simulink model "IRGLMHybridController"  (R2022b)
settings: Solver=FixedStepAuto  StartTime=0.0  StopTime=1E6  FixedStep=1/2000  RelTol=1e-3
undefined symbols (not defined in the file): Pull, up
libraries: cstblocks x7, speedgoatlib_IO183 x5, slrealtimeutilitieslib x2, slrealtimeiplib x2, dspstat3 x1
settings Model: Creator=MOSA  LastModifiedBy=MOSA
settings SolverCC: ConcurrentTasks=on  PositivePriorityOrder=on
settings OptimizationCC: BlockReduction=off  OptimizeBlockIOStorage=off
settings DebuggingCC: TasksWithSamePriorityMsg=none
settings HardwareCC: ProdBitPerLong=64  ProdLongLongMode=on  ProdHWDeviceType=Intel->x86-64 (Linux 64)
settings RTWCC: Description=Simulink Real-Time  SystemTargetFile=slrealtime.tlc  TemplateMakefile=slrealtime_default_tmf  Toolchain=Simulink Real-Time Toolchain  BuildConfiguration=Faster Runs  CodeExecutionProfiling=on  TargetLang=C++

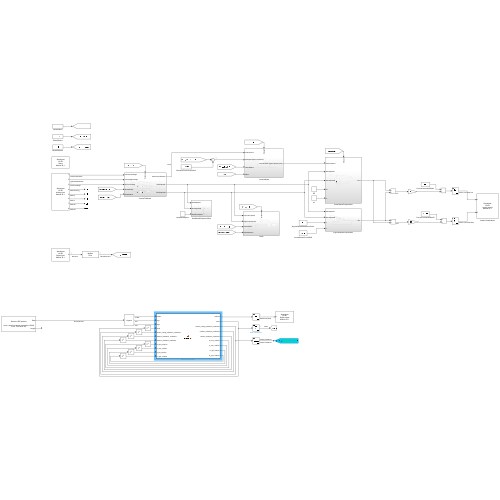
[thumbnail: Simulink's stored preview of the top-level diagram]
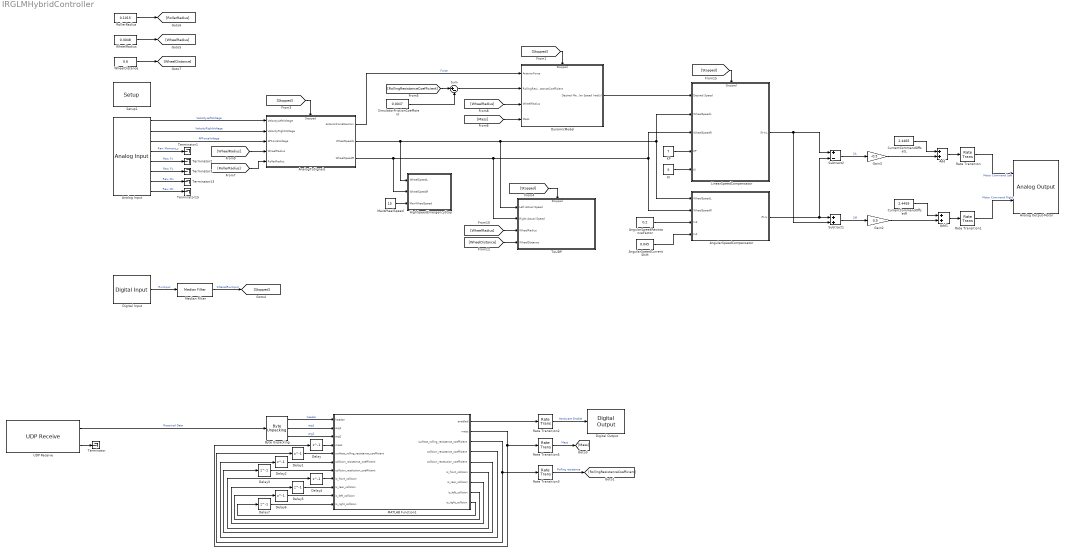
== system IRGLMHybridController ==
  Add : Sum
  Add1 : Sum
  Analog Input : speedgoatlib_IO183/Analog Input  Priority=0  parModuleId=1  parSampTime=1/2000  parPciSlot=-1  parAdChannelLow=1  parAdChannelHigh=8
      settings: SourceProductName=Simulink Real-Time: Speedgoat I/O Blockset
  Analog Output-Motor : speedgoatlib_IO183/Analog Output  parModuleId=1  parSampTime=-1  parDaSimult=on  parPciSlot=-1  parDaChannels=[1 2]  parDaInit=[0 0 0 0]  parDaReset=[1 1 1 1]
      settings: SourceProductName=Simulink Real-Time: Speedgoat I/O Blockset
  AnalogToSignals : Subsystem
      settings: PortSchema="{\"entries\":[{\"content\":{\"sides\":[{\"content\":{\"connectorIds\":[\"In1\",\"In2\",\"In3\",\"In4\",\"In5\"]},\"type\":\"ConnectorPlacement.EquallySpacedRectSide\",\"uuid\":\"33d34f65-8288-4f26-a259-c6a495dc8706\"},{\"content\":{\"connectorIds\":[\"Out1\",\"Out2\",\"Out3\"],\"side\":\"RIGHT\"},\"type\":\"ConnectorPlacement.EquallySpacedRectSide\",\"uuid\":\"464c1a73-e25a-412b-b070-c0497a01c93b\"},{\"content\":{\"connectorIds\":[\"In6\"],\"side\":\"TOP\"},\"type\":\"ConnectorPlacement.EquallySpacedRectSide\",\"uuid\":\"eb57de37-2540-4fa6-8c21-04ed7dfe5e59\"}]},\"type\":\"ConnectorPlacement.EquallySpacedConnector\",\"uuid\":\"7b998d75-753a-4c6e-bb60-3204e0b4afb9\"}],\"packageUris\":[\"http://schema.mathworks.com/mf0/Connector/R2020b\"],\"version\":\"1.0\"}"
  AngularSpeedCompensator : Subsystem
  AngularSpeedCurrentShift : Constant  Value=0.045
  AngularSpeedResistanceFactor : Constant  Value=0.2
  Byte Unpacking : slrealtimeutilitieslib/Byte Unpacking  MaskUnpackedDataTypes={['uint32'],['double'],['double']}  MaskUnpackedDataSizes={[1] [1] [1]}  MaskAlignment=4
  CurrentCommandOffsetL : Constant  Value=2.4465
  CurrentCommandOffsetR : Constant  Value=2.4459
  Delay{,1..7} (8 alike) : Delay  DelayLength=1  InitialCondition=0
  Digital Input : speedgoatlib_IO183/Digital Input  parModuleId=1  parSampTime=1/2000  parPciSlot=-1  parDiChannels=2
      settings: SourceProductName=Simulink Real-Time: Speedgoat I/O Blockset
  Digital Output : speedgoatlib_IO183/Digital Output  parModuleId=1  parSampTime=-1  parPciSlot=-1  parDoChannels=1  parDoInit=0  parDoReset=1
      settings: SourceProductName=Simulink Real-Time: Speedgoat I/O Blockset
  DynamicModel : Subsystem
      settings: PortSchema="{\"entries\":[{\"content\":{\"sides\":[{\"content\":{\"connectorIds\":[\"In1\",\"In2\",\"In3\",\"In4\"]},\"type\":\"ConnectorPlacement.EquallySpacedRectSide\",\"uuid\":\"698b5f1b-e41d-47ec-8a78-8e111d48540c\"},{\"content\":{\"connectorIds\":[\"Out1\"],\"side\":\"RIGHT\"},\"type\":\"ConnectorPlacement.EquallySpacedRectSide\",\"uuid\":\"a52a2d34-ec8e-4f9e-8684-ea9d86dd283b\"},{\"content\":{\"connectorIds\":[\"In5\"],\"side\":\"TOP\"},\"type\":\"ConnectorPlacement.EquallySpacedRectSide\",\"uuid\":\"faf14a61-efdc-45c6-85a8-2f82d0ccb291\"}]},\"type\":\"ConnectorPlacement.EquallySpacedConnector\",\"uuid\":\"7a7495df-049f-4dbe-8bcc-a94b4d420872\"}],\"packageUris\":[\"http://schema.mathworks.com/mf0/Connector/R2020b\"],\"version\":\"1.0\"}"
  Gain2 : Gain  Gain=0.5
  Gain3 : Gain  Gain=-0.5
  HighSpeedEmergencyStop : Subsystem
  KI : Constant  Value=5
  KP : Constant  Value=7
  LinearSpeedCompensator : Subsystem
      settings: PortSchema="{\"entries\":[{\"content\":{\"sides\":[{\"content\":{\"connectorIds\":[\"In1\",\"In2\",\"In3\",\"In4\",\"In5\"]},\"type\":\"ConnectorPlacement.EquallySpacedRectSide\",\"uuid\":\"9b7edc03-5e72-48f4-bed7-21920e73c297\"},{\"content\":{\"connectorIds\":[\"Out1\"],\"side\":\"RIGHT\"},\"type\":\"ConnectorPlacement.EquallySpacedRectSide\",\"uuid\":\"1856f1b7-fc85-471c-9138-bfce3ff137ef\"},{\"content\":{\"connectorIds\":[\"In6\"],\"side\":\"TOP\"},\"type\":\"ConnectorPlacement.EquallySpacedRectSide\",\"uuid\":\"701dcd4a-e839-44a9-b16d-b7c230713f8d\"}]},\"type\":\"ConnectorPlacement.EquallySpacedConnector\",\"uuid\":\"564dc47d-1095-4697-b7b0-537dc9d65b40\"}],\"packageUris\":[\"http://schema.mathworks.com/mf0/Connector/R2020b\"],\"version\":\"1.0\"}"
  MATLAB Function1 : MATLAB Function  TreatAsAtomicUnit=on
  MaxWheelSpeed : Constant  Value=15
  Median Filter : dspstat3/Median Filter  WindowLength=5  SimulateUsing=Interpreted execution
      settings: LibrarySourceBlock=|
      | dspfdesign/Median
      | Filter
  Rate Transition : RateTransition
  Rate Transition1 : RateTransition
  Rate Transition2 : RateTransition  OutPortSampleTime=1/2000
  Rate Transition3 : RateTransition  OutPortSampleTime=1/2000
  Rate Transition5 : RateTransition  OutPortSampleTime=1/2000
  RollerRadius : Constant  Value=0.1015
  Setup1 : speedgoatlib_IO183/Setup  parModuleId=1  parPciSlot=-1  parDaSimult=on  parAdCoupling=Single Ended  parAdRange=+-10V  parAdChannelLow=1  parAdChannelHigh=8  parDaChannels=[1:2]  parDaRange=0..5V  parDaInit=[0]  parDaReset=[1]  parDoChannels=[1]  parDoInit=[0]  parDoReset=[1]  parDiChannels=[2]  parIOPullReferenceFront=Pull-up (3.3V)  parIOPullReferenceRear=Pull-up (3.3V)
      settings: SourceProductName=Simulink Real-Time: Speedgoat I/O Blockset
  SimulatorFrictionCoefficient : Constant  Value=0.0047
  Subtract1 : Sum
  Subtract2 : Sum  Inputs=+-
  Sum : Sum  Inputs=|+-
  Terminator{,1..3,13,15} (6 alike) : Terminator
  ToUDP : Subsystem
      settings: PortSchema="{\"entries\":[{\"content\":{\"sides\":[{\"content\":{\"connectorIds\":[\"In1\",\"In2\",\"In3\",\"In4\"]},\"type\":\"ConnectorPlacement.EquallySpacedRectSide\",\"uuid\":\"20cbcfc2-0ca7-4a2f-a613-0278f24034ac\"},{\"content\":{\"connectorIds\":[],\"side\":\"RIGHT\"},\"type\":\"ConnectorPlacement.EquallySpacedRectSide\",\"uuid\":\"dd88a308-46d9-424c-b176-6f22faf13019\"},{\"content\":{\"connectorIds\":[\"In5\"],\"side\":\"TOP\"},\"type\":\"ConnectorPlacement.EquallySpacedRectSide\",\"uuid\":\"69795427-50da-496d-bb46-4af6bccb20c3\"},{\"content\":{\"connectorIds\":[],\"side\":\"BOTTOM\"},\"type\":\"ConnectorPlacement.EquallySpacedRectSide\",\"uuid\":\"b34d6e53-d8ac-4a7b-a484-2036578c791d\"}]},\"type\":\"ConnectorPlacement.EquallySpacedConnector\",\"uuid\":\"611fc7d8-fafd-42e7-a535-d43e2501456a\"}],\"packageUris\":[\"http://schema.mathworks.com/mf0/Connector/R2020b\"],\"version\":\"1.0\"}"
  UDP Receive : slrealtimeiplib/UDP Receive  useHostTargetConn=on  ipAddress=192.168.0.200  localPort=25000  rcvWidth=20  rcvFmAny=off  fmAddress=192.168.0.159  sampleTime=1/200  enableMessage=off  maxPackets=1
  WheelDistance : Constant  Value=0.6
  WheelRadius : Constant  Value=0.3048
  wires:
  KI/1 -> LinearSpeedCompensator/5(KI)
  [Stopped] -> ToUDP/5(Stopped)
  [RollingResistanceCoefficient] -> Sum/1
  Subtract1/1 -> Gain2/1  "2iR"
  Sum/1 -> DynamicModel/2(RollingResistanceCoefficient)
  Gain3/1 -> Add/2
  Gain2/1 -> Add1/2
  Analog Input/5 -> Terminator2/1  "Raw Fx"
  Rate Transition1/1 -> Analog Output-Motor/2  "Motor Command Right"
  DynamicModel/1(Desired Mean Angular Speed (rad/s)) -> LinearSpeedCompensator/1(Desired Speed)
  KP/1 -> LinearSpeedCompensator/4(KP)
  [Stopped] -> LinearSpeedCompensator/6(Stopped)
  LinearSpeedCompensator/1(iR+iL) -> Subtract2/1, Subtract1/2
  UDP Receive/1 -> Byte Unpacking/1  "Received Data"
  Rate Transition2/1 -> Digital Output/1  "Hardware Enable"
  Digital Input/1 -> Median Filter/1  "RunInput"
  SimulatorFrictionCoefficient/1 -> Sum/2
  Analog Input/4 -> Terminator1/1  "Raw Moment_y"
  Median Filter/1 -> [Stopped]  "FilteredRunInput"
  Analog Input/7 -> Terminator13/1  "Raw Mx"
  Analog Input/6 -> Terminator3/1  "Raw Fy"
  Analog Input/8 -> Terminator15/1  "Raw Mz"
  UDP Receive/2 -> Terminator/1
  AnalogToSignals/1(AnteriorForceNewton) -> DynamicModel/1("AnteriorForce ")  "Force"
  Rate Transition/1 -> Analog Output-Motor/1  "Motor Command Left"
  Subtract2/1 -> Gain3/1  "2iL"
  Add/1 -> Rate Transition/1
  CurrentCommandOffsetR/1 -> Add1/1
  Rate Transition5/1 -> [Mass]  "Mass"
  Rate Transition3/1 -> [RollingResistanceCoefficient]  "Rolling resistance"
  CurrentCommandOffsetL/1 -> Add/1
  Add1/1 -> Rate Transition1/1
  [Mass] -> DynamicModel/4(Mass)
  WheelRadius/1 -> [WheelRadius]
  [WheelDistance] -> ToUDP/4(WheelDistance)
  RollerRadius/1 -> [RollerRadius]
  [WheelRadius] -> DynamicModel/3(WheelRadius)
  [WheelRadius] -> ToUDP/3(WheelRadius)
  WheelDistance/1 -> [WheelDistance]
  AnalogToSignals/2(WheelSpeedL) -> HighSpeedEmergencyStop/1(WheelSpeedL), AngularSpeedCompensator/1(WheelSpeedL), LinearSpeedCompensator/2(WheelSpeedL), ToUDP/1(Left Actual Speed)
  AnalogToSignals/3(WheelSpeedR) -> HighSpeedEmergencyStop/2(WheelSpeedR), LinearSpeedCompensator/3(WheelSpeedR), AngularSpeedCompensator/2(WheelSpeedR), ToUDP/2(Right Actual Speed)
  Analog Input/1 -> AnalogToSignals/1(VelocityLeftVoltage)  "VelocityLeftVoltage"
  Analog Input/2 -> AnalogToSignals/2(VelocityRightVoltage)  "VelocityRightVoltage"
  Analog Input/3 -> AnalogToSignals/3(APForceVoltage)  "APForceVoltage"
  [WheelRadius] -> AnalogToSignals/4(WheelRadius)
  [RollerRadius] -> AnalogToSignals/5(RollerRadius)
  [Stopped] -> AnalogToSignals/6(Stopped)
  [Stopped] -> DynamicModel/5(Stopped)
  MaxWheelSpeed/1 -> HighSpeedEmergencyStop/3(MaxWheelSpeed)
  AngularSpeedCompensator/1(iR-iL) -> Subtract1/1, Subtract2/2
  AngularSpeedResistanceFactor/1 -> AngularSpeedCompensator/3(In3)
  AngularSpeedCurrentShift/1 -> AngularSpeedCompensator/4(In4)
  Byte Unpacking/1 -> MATLAB Function1/1(header)  "header"
  Byte Unpacking/2 -> MATLAB Function1/2(arg1)  "arg1"
  Byte Unpacking/3 -> MATLAB Function1/3(arg2)  "arg2"
  MATLAB Function1/1(enabled) -> Rate Transition2/1
  MATLAB Function1/9(is_right_collision) -> Delay7/1
  MATLAB Function1/8(is_left_collision) -> Delay6/1
  MATLAB Function1/7(is_rear_collision) -> Delay5/1
  MATLAB Function1/6(is_front_collision) -> Delay4/1
  MATLAB Function1/5(collision_restitution_coefficient) -> Delay3/1
  MATLAB Function1/4(collision_resistance_coefficient) -> Delay2/1
  MATLAB Function1/3(surface_rolling_resistance_coefficient) -> Rate Transition3/1, Delay1/1
  MATLAB Function1/2(mass) -> Rate Transition5/1, Delay/1
  Delay/1 -> MATLAB Function1/4("mass ")
  Delay1/1 -> MATLAB Function1/5("surface_rolling_resistance_coefficient ")
  Delay2/1 -> MATLAB Function1/6("collision_resistance_coefficient ")
  Delay3/1 -> MATLAB Function1/7("collision_restitution_coefficient ")
  Delay4/1 -> MATLAB Function1/8("is_front_collision ")
  Delay5/1 -> MATLAB Function1/9("is_rear_collision ")
  Delay6/1 -> MATLAB Function1/10("is_left_collision ")
  Delay7/1 -> MATLAB Function1/11("is_right_collision ")

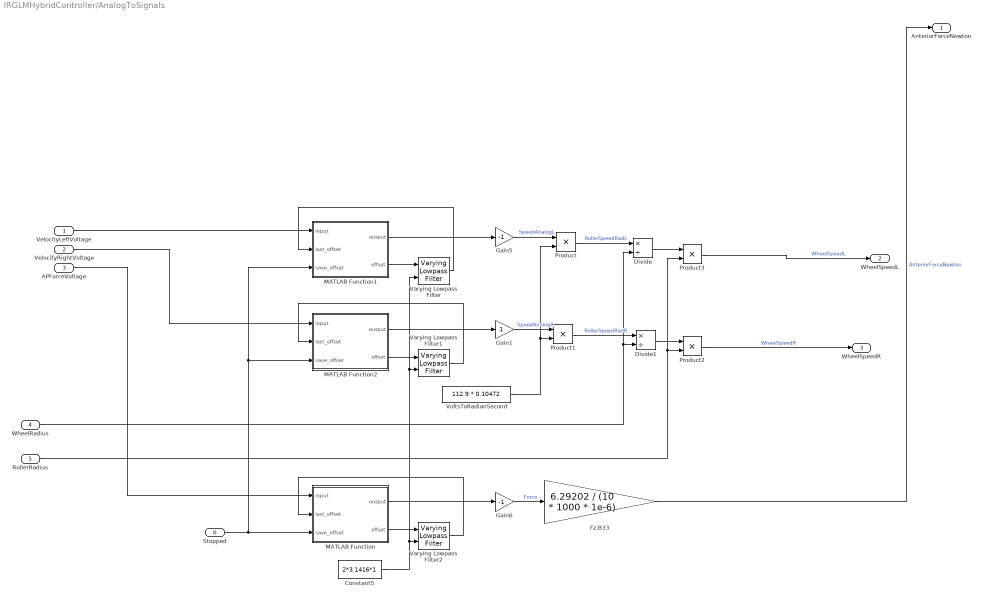
== system IRGLMHybridController/AnalogToSignals ==
  VelocityLeftVoltage : Inport
  VelocityRightVoltage : Inport  Port=2
  APForceVoltage : Inport  Port=3
  WheelRadius : Inport  Port=4
  RollerRadius : Inport  Port=5
  Stopped : Inport  Port=6
  Constant5 : Constant  Value=2*3.1416*1
  Divide : Product  Inputs=*/
  Divide1 : Product  Inputs=*/
  Fz.B33 : Gain  Gain="6.29202 / (10 * 1000  * 1e-6)"
  Gain1 : Gain
  Gain5 : Gain  Gain=-1
  Gain6 : Gain  Gain=-1
  MATLAB Function : MATLAB Function  TreatAsAtomicUnit=on
  MATLAB Function1 : MATLAB Function  TreatAsAtomicUnit=on
  MATLAB Function2 : MATLAB Function  TreatAsAtomicUnit=on
  Product{,1..3} (4 alike) : Product
  Varying Lowpass Filter : cstblocks/Linear Parameter Varying/Varying Lowpass Filter  N=1
  Varying Lowpass Filter1 : cstblocks/Linear Parameter Varying/Varying Lowpass Filter  N=1
  Varying Lowpass Filter2 : cstblocks/Linear Parameter Varying/Varying Lowpass Filter  N=1
  VoltsToRadianSecond : Constant  Value=112.9 * 0.10472
  AnteriorForceNewton : Outport
  WheelSpeedL : Outport  Port=2
  WheelSpeedR : Outport  Port=3
  wires:
  VelocityLeftVoltage/1 -> MATLAB Function1/1(input)
  Stopped/1 -> MATLAB Function1/3(save_offset), MATLAB Function2/3(save_offset), MATLAB Function/3(save_offset)
  WheelRadius/1 -> Divide/2, Divide1/2
  Gain5/1 -> Product/1  "SpeedAnalogL"
  Product2/1 -> WheelSpeedR/1  "WheelSpeedR"
  MATLAB Function1/2(offset) -> Varying Lowpass Filter/1
  Constant5/1 -> Varying Lowpass Filter/2, Varying Lowpass Filter1/2, Varying Lowpass Filter2/2
  Varying Lowpass Filter1/1 -> MATLAB Function2/2(last_offset)
  Product3/1 -> WheelSpeedL/1  "WheelSpeedL"
  Varying Lowpass Filter/1 -> MATLAB Function1/2(last_offset)
  RollerRadius/1 -> Product3/2, Product2/2
  VoltsToRadianSecond/1 -> Product/2, Product1/2
  MATLAB Function1/1(output) -> Gain5/1
  MATLAB Function2/1(output) -> Gain1/1
  Product1/1 -> Divide1/1  "RollerSpeedRadR"
  Gain1/1 -> Product1/1  "SpeedAnalogR"
  Product/1 -> Divide/1  "RollerSpeedRadL"
  MATLAB Function2/2(offset) -> Varying Lowpass Filter1/1
  MATLAB Function/1(output) -> Gain6/1
  Gain6/1 -> Fz.B33/1  "Force"
  MATLAB Function/2(offset) -> Varying Lowpass Filter2/1
  Divide1/1 -> Product2/1
  Fz.B33/1 -> AnteriorForceNewton/1  "AnteriorForceNewton"
  Divide/1 -> Product3/1
  APForceVoltage/1 -> MATLAB Function/1(input)
  Varying Lowpass Filter2/1 -> MATLAB Function/2(last_offset)
  VelocityRightVoltage/1 -> MATLAB Function2/1(input)

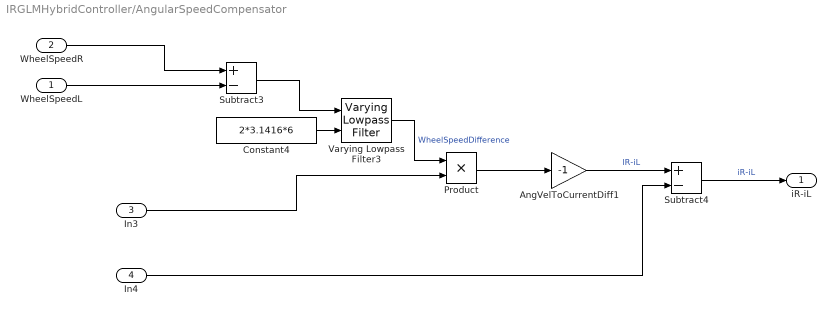
== system IRGLMHybridController/AngularSpeedCompensator ==
  WheelSpeedL : Inport
  WheelSpeedR : Inport  Port=2
  In3 : Inport  Port=3
  In4 : Inport  Port=4
  AngVelToCurrentDiff1 : Gain  Gain=-1
  Constant4 : Constant  Value=2*3.1416*6
  Product : Product
  Subtract3 : Sum  Inputs=+-
  Subtract4 : Sum  Inputs=+-
  Varying Lowpass Filter3 : cstblocks/Linear Parameter Varying/Varying Lowpass Filter  N=2
  iR-iL : Outport
  wires:
  Varying Lowpass Filter3/1 -> Product/1  "WheelSpeedDifference"
  Subtract3/1 -> Varying Lowpass Filter3/1
  AngVelToCurrentDiff1/1 -> Subtract4/1  "lR-iL"
  In3/1 -> Product/2
  Constant4/1 -> Varying Lowpass Filter3/2
  Product/1 -> AngVelToCurrentDiff1/1
  WheelSpeedL/1 -> Subtract3/2
  Subtract4/1 -> iR-iL/1  "iR-iL"
  In4/1 -> Subtract4/2
  WheelSpeedR/1 -> Subtract3/1

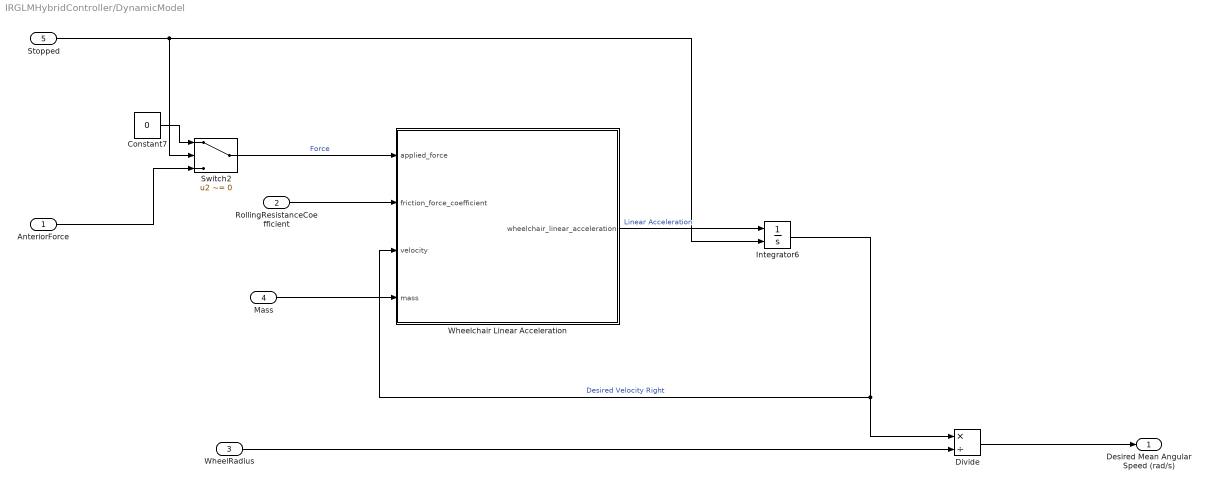
== system IRGLMHybridController/DynamicModel ==
  "AnteriorForce " : Inport
  RollingResistanceCoefficient : Inport  Port=2
  WheelRadius : Inport  Port=3
  Mass : Inport  Port=4
  Stopped : Inport  Port=5
  Constant7 : Constant  Value=0
  Divide : Product  Inputs=*/
  Integrator6 : Integrator  ExternalReset=level hold
  Switch2 : Switch  Criteria=u2 ~= 0  SaturateOnIntegerOverflow=off  InputSameDT=off
  Wheelchair Linear Acceleration : MATLAB Function  TreatAsAtomicUnit=on
  Desired Mean Angular Speed (rad/s) : Outport
  wires:
  Divide/1 -> Desired Mean Angular Speed (rad/s)/1
  Mass/1 -> Wheelchair Linear Acceleration/4(mass)
  Integrator6/1 -> Divide/1, Wheelchair Linear Acceleration/3(velocity)  "Desired Velocity Right"
  RollingResistanceCoefficient/1 -> Wheelchair Linear Acceleration/2(friction_force_coefficient)
  WheelRadius/1 -> Divide/2
  Wheelchair Linear Acceleration/1(wheelchair_linear_acceleration) -> Integrator6/1  "Linear Acceleration"
  Constant7/1 -> Switch2/1
  "AnteriorForce "/1 -> Switch2/3
  Switch2/1 -> Wheelchair Linear Acceleration/1(applied_force)  "Force"
  Stopped/1 -> Integrator6/2, Switch2/2

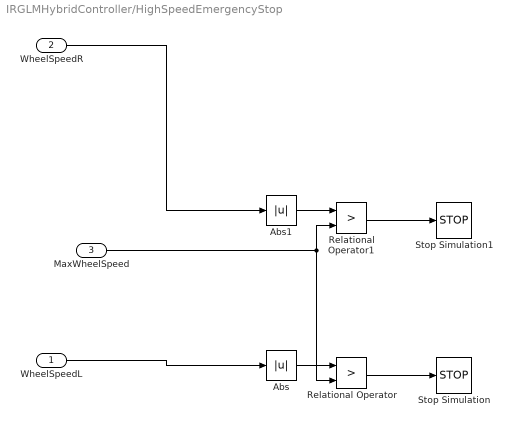
== system IRGLMHybridController/HighSpeedEmergencyStop ==
  WheelSpeedL : Inport
  WheelSpeedR : Inport  Port=2
  MaxWheelSpeed : Inport  Port=3
  Abs : Abs  SaturateOnIntegerOverflow=off
  Abs1 : Abs  SaturateOnIntegerOverflow=off
  Relational Operator : RelationalOperator  Operator=>  OutDataTypeStr=boolean  RndMeth=Simplest  InputSameDT=off
  Relational Operator1 : RelationalOperator  Operator=>  OutDataTypeStr=boolean  RndMeth=Simplest  InputSameDT=off
  Stop Simulation : Stop
  Stop Simulation1 : Stop
  wires:
  MaxWheelSpeed/1 -> Relational Operator/2, Relational Operator1/2
  Relational Operator/1 -> Stop Simulation/1
  WheelSpeedR/1 -> Abs1/1
  WheelSpeedL/1 -> Abs/1
  Abs/1 -> Relational Operator/1
  Relational Operator1/1 -> Stop Simulation1/1
  Abs1/1 -> Relational Operator1/1

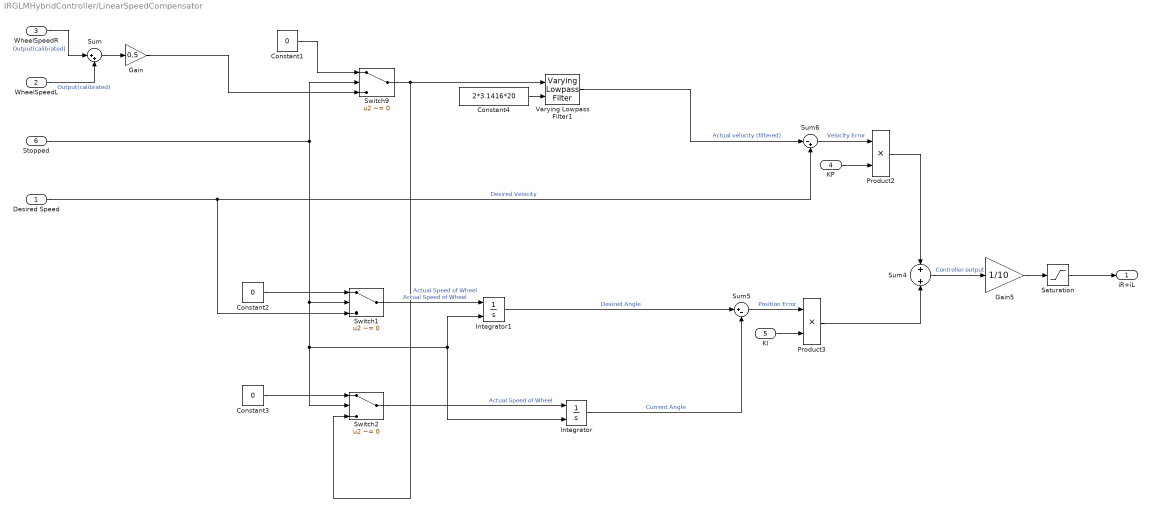
== system IRGLMHybridController/LinearSpeedCompensator ==
  Desired Speed : Inport
  WheelSpeedL : Inport  Port=2
  WheelSpeedR : Inport  Port=3
  KP : Inport  Port=4
  KI : Inport  Port=5
  Stopped : Inport  Port=6
  Constant1 : Constant  Value=0
  Constant2 : Constant  Value=0
  Constant3 : Constant  Value=0
  Constant4 : Constant  Value=2*3.1416*20
  Gain : Gain  Gain=0.5
  Gain5 : Gain  Gain=1/10
  Integrator : Integrator  ExternalReset=level hold
  Integrator1 : Integrator  ExternalReset=level hold
  Product2 : Product  RndMeth=Zero
  Product3 : Product  RndMeth=Zero
  Saturation : Saturate  UpperLimit=4  LowerLimit=-4
  Sum : Sum  Inputs=|++
  Sum4 : Sum
  Sum5 : Sum  Inputs=|+-
  Sum6 : Sum  Inputs=|-+
  Switch1 : Switch  Criteria=u2 ~= 0  SaturateOnIntegerOverflow=off  InputSameDT=off
  Switch2 : Switch  Criteria=u2 ~= 0  SaturateOnIntegerOverflow=off  InputSameDT=off
  Switch9 : Switch  Criteria=u2 ~= 0  SaturateOnIntegerOverflow=off  InputSameDT=off
  Varying Lowpass Filter1 : cstblocks/Linear Parameter Varying/Varying Lowpass Filter  N=2
  iR+iL : Outport
  wires:
  Varying Lowpass Filter1/1 -> Sum6/1  "Actual velocity (filtered)"
  Product2/1 -> Sum4/1
  Sum5/1 -> Product3/1  "Position Error"
  KP/1 -> Product2/2
  Stopped/1 -> Switch9/2, Switch1/2, Integrator/2, Integrator1/2, Switch2/2
  Gain5/1 -> Saturation/1
  Switch9/1 -> Switch2/3, Varying Lowpass Filter1/1  "Actual Speed of Wheel"
  Desired Speed/1 -> Switch1/3, Sum6/2  "Desired Velocity"
  Sum4/1 -> Gain5/1  "Controller output"
  Integrator/1 -> Sum5/2  "Current Angle"
  Integrator1/1 -> Sum5/1  "Desired Angle"
  Saturation/1 -> iR+iL/1
  Sum6/1 -> Product2/1  "Velocity Error"
  KI/1 -> Product3/2
  Product3/1 -> Sum4/2
  Sum/1 -> Gain/1
  Gain/1 -> Switch9/3
  Constant1/1 -> Switch9/1
  WheelSpeedR/1 -> Sum/1  "Output(calibrated)"
  WheelSpeedL/1 -> Sum/2  "Output(calibrated)"
  Constant2/1 -> Switch1/1
  Constant3/1 -> Switch2/1
  Switch1/1 -> Integrator1/1  "Actual Speed of Wheel"
  Switch2/1 -> Integrator/1  "Actual Speed of Wheel"
  Constant4/1 -> Varying Lowpass Filter1/2

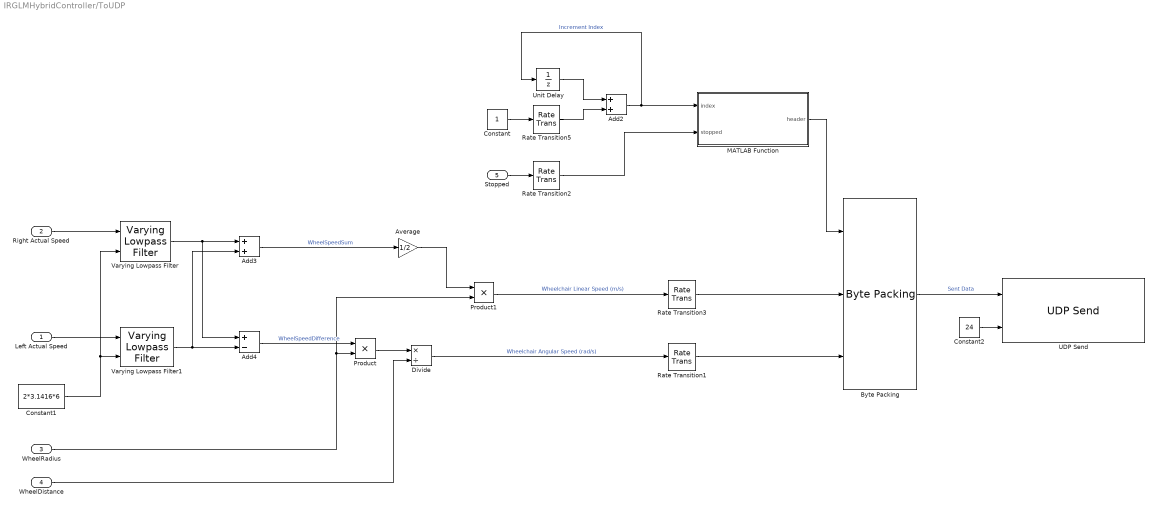
== system IRGLMHybridController/ToUDP ==
  Left Actual Speed : Inport
  Right Actual Speed : Inport  Port=2
  WheelRadius : Inport  Port=3
  WheelDistance : Inport  Port=4
  Stopped : Inport  Port=5
  Add2 : Sum
  Add3 : Sum
  Add4 : Sum  Inputs=+-
  Average : Gain  Gain=1/2
  Byte Packing : slrealtimeutilitieslib/Byte Packing  MaskPackedDataType=uint8  MaskUnpackedDataTypes={['uint32'],['double'],['double']}  MaskAlignment=1
  Constant : Constant
  Constant1 : Constant  Value=2*3.1416*6
  Constant2 : Constant  Value=24
  Divide : Product  Inputs=*/
  MATLAB Function : MATLAB Function  TreatAsAtomicUnit=on
  Product : Product
  Product1 : Product
  Rate Transition{1..3,5} (4 alike) : RateTransition  OutPortSampleTime=1/50
  UDP Send : slrealtimeiplib/UDP Send  useHostTargetConn=on  toAddress=192.168.0.159  toPort=25100  sampleTime=-1  enableMessage=off  ipAddress=192.168.0.200  localPort=25000
  Unit Delay : UnitDelay  SampleTime=-1  HasFrameUpgradeWarning=on
  Varying Lowpass Filter : cstblocks/Linear Parameter Varying/Varying Lowpass Filter  N=1
  Varying Lowpass Filter1 : cstblocks/Linear Parameter Varying/Varying Lowpass Filter  N=1
  wires:
  Varying Lowpass Filter/1 -> Add3/1, Add4/1
  Unit Delay/1 -> Add2/1
  Divide/1 -> Rate Transition1/1  "Wheelchair Angular Speed (rad/s)"
  Add2/1 -> MATLAB Function/1(index), Unit Delay/1  "Increment Index"
  Constant/1 -> Rate Transition5/1
  Product1/1 -> Rate Transition3/1  "Wheelchair Linear Speed (m/s)"
  Add3/1 -> Average/1  "WheelSpeedSum"
  Varying Lowpass Filter1/1 -> Add4/2, Add3/2
  Right Actual Speed/1 -> Varying Lowpass Filter/1
  Left Actual Speed/1 -> Varying Lowpass Filter1/1
  Constant1/1 -> Varying Lowpass Filter/2, Varying Lowpass Filter1/2
  Product/1 -> Divide/1
  Add4/1 -> Product/1  "WheelSpeedDifference"
  WheelRadius/1 -> Product1/2, Product/2
  WheelDistance/1 -> Divide/2
  Average/1 -> Product1/1
  Constant2/1 -> UDP Send/2
  Byte Packing/1 -> UDP Send/1  "Sent Data"
  Rate Transition5/1 -> Add2/2
  Stopped/1 -> Rate Transition2/1
  Rate Transition2/1 -> MATLAB Function/2(stopped)
  MATLAB Function/1(header) -> Byte Packing/1
  Rate Transition3/1 -> Byte Packing/2
  Rate Transition1/1 -> Byte Packing/3

== matlab function IRGLMHybridController/MATLAB Function1 ==
  data: enabled output; header input; arg1 input; arg2 input; mass output; mass input; surface_rolling_resistance_coefficient input; surface_rolling_resistance_coefficient output; collision_resistance_coefficient input; collision_restitution_coefficient input; is_front_collision input; is_rear_collision input; is_left_collision input; is_right_collision input; collision_resistance_coefficient output; collision_restitution_coefficient output; is_front_collision output; is_rear_collision output; is_left_collision output; is_right_collision output
function [ ...
    enabled, ...
    mass, ...
    surface_rolling_resistance_coefficient, ...
    collision_resistance_coefficient, ...
    collision_restitution_coefficient, ...
    is_front_collision, ...
    is_rear_collision, ...
    is_left_collision, ...
    is_right_collision ...
] = receivedata( ...
    header, ...
    arg1, ...
    arg2, ...
    mass, ...
    surface_rolling_resistance_coefficient, ...
    collision_resistance_coefficient, ...
    collision_restitution_coefficient, ...
    is_front_collision, ...
    is_rear_collision, ...
    is_left_collision, ...
    is_right_collision ...
)

    header = uint32(header);
    cmd = mod(uint32(header / 2^16), 2^12);
    enabled = double(mod(header, 2));

    switch(cmd)
        case 1 % Inertia update
            mass = arg1;
        case 2 % Surface rolling resistance update
            surface_rolling_resistance_coefficient = arg1;
        case 3 % Front collision enter
            collision_resistance_coefficient = arg1;
            collision_restitution_coefficient = arg2;
            is_front_collision = 1;
        case 4 % Front collision exit
            is_front_collision = 0;
        case 5 % Rear collision enter
            collision_resistance_coefficient = arg1;
            collision_restitution_coefficient = arg2;
            is_rear_collision = 1;
        case 6 % Rear collision exit
            is_rear_collision = 0;
        case 7 % Left collision enter
            collision_resistance_coefficient = arg1;
            collision_restitution_coefficient = arg2;
            is_left_collision = 1;
        case 8 % Left collision exit
            is_left_collision = 0;
        case 9 % Right collision enter
            collision_resistance_coefficient = arg1;
            collision_restitution_coefficient = arg2;
            is_right_collision = 1;
        case 10 % Front collision exit
            is_right_collision = 0;
    end


end

== matlab function IRGLMHybridController/ToUDP/MATLAB Function ==
  data: index input; header output; stopped input
function header = createheader(index, stopped)

index = mod(index, 16);
command = 1;  % Speed Update
stopped = boolean(stopped);
state = stopped;

header = uint32(index * (2^28) + command * (2^16) + state);

== matlab function IRGLMHybridController/AnalogToSignals/MATLAB Function ==
  data: input input; output output; last_offset input; save_offset input; offset output
function [output, offset]= remove_offset(input, last_offset, save_offset)
    if save_offset > 0
        offset = input;
    else
        offset = last_offset;
    end
    output = input - offset;
end

== matlab function IRGLMHybridController/AnalogToSignals/MATLAB Function1 ==
  data: input input; output output; last_offset input; save_offset input; offset output
function [output, offset]= remove_offset(input, last_offset, save_offset)
    if save_offset > 0
        offset = input;
    else
        offset = last_offset;
    end
    output = input - offset;
end

== matlab function IRGLMHybridController/AnalogToSignals/MATLAB Function2 ==
  data: input input; output output; last_offset input; save_offset input; offset output
function [output, offset]= remove_offset(input, last_offset, save_offset)
    if save_offset > 0
        offset = input;
    else
        offset = last_offset;
    end
    output = input - offset;
end

== matlab function IRGLMHybridController/DynamicModel/Wheelchair Linear Acceleration ==
  data: applied_force input; friction_force_coefficient input; velocity input; wheelchair_linear_acceleration output; mass input
function wheelchair_linear_acceleration  = wheelchair_linear(applied_force, friction_force_coefficient, velocity, mass)

if mass < 1  % Uninitialized yet, avoid a 0/0 indetermination
    mass = 1;
end

g = 9.81;

friction_force = friction_force_coefficient*mass*g;
sum_of_forces = (applied_force - friction_force * sign(velocity));
wheelchair_linear_acceleration = sum_of_forces / mass;
